simulink model "FighterAC"  (R2018a)
settings: Solver=ode2  StartTime=0.0  StopTime=T_final  FixedStep=dt_sim  RelTol=1e-3
undefined symbols (not defined in the file): b, Cl_da, Cl_dr, Cl_p, Cl_r, Cn_da, Cn_dr, Cn_p, Cn_r, Cy_da, Cy_dr, Cy_p, Cy_r, g, Ixx, Izz, mass, S_ref, V_ini
libraries: simulink_need_slupdate x4
settings Model: Creator=Can  LastModifiedBy=Can

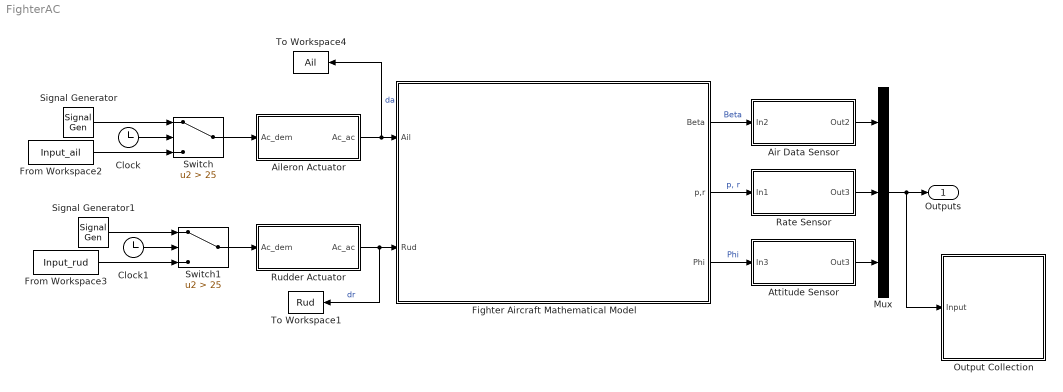
== system FighterAC ==
  Aileron Actuator : Subsystem
  Air Data Sensor : Subsystem
  Attitude Sensor : Subsystem
  Clock : Clock
  Clock1 : Clock
  Fighter Aircraft Mathematical Model : Subsystem
      mask Display: image('C:\Users\Can\Desktop\Thesis_v3\MMU.PNG')
  From Workspace2 : FromWorkspace  VariableName=Input_ail  SampleTime=0
  From Workspace3 : FromWorkspace  VariableName=Input_rud  SampleTime=0
  Mux : Mux  Inputs=3
  "Output Collection " : Subsystem
  Rate Sensor : Subsystem
  Rudder Actuator : Subsystem
  Signal Generator : SignalGenerator  WaveForm=square  Amplitude=0.05  Units=rad/sec
  Signal Generator1 : SignalGenerator  WaveForm=square  Amplitude=0.05  Units=rad/sec
  Switch : Switch  Criteria=u2 > Threshold  Threshold=25
  Switch1 : Switch  Criteria=u2 > Threshold  Threshold=25
  To Workspace1 : ToWorkspace  VariableName=Rud  SaveFormat=Structure With Time  SampleTime=-1
  To Workspace4 : ToWorkspace  VariableName=Ail  SaveFormat=Structure With Time  SampleTime=-1
  Outputs : Outport
  wires:
  From Workspace2/1 -> Switch/3
  Clock/1 -> Switch/2
  Signal Generator/1 -> Switch/1
  Signal Generator1/1 -> Switch1/1
  Clock1/1 -> Switch1/2
  From Workspace3/1 -> Switch1/3
  Attitude Sensor/1(Out3) -> Mux/3
  Air Data Sensor/1(Out2) -> Mux/1
  Fighter Aircraft Mathematical Model/3(Phi) -> Attitude Sensor/1(In3)  "Phi"
  Fighter Aircraft Mathematical Model/1(Beta) -> Air Data Sensor/1(In2)  "Beta"
  Rudder Actuator/1(Ac_ac) -> To Workspace1/1, Fighter Aircraft Mathematical Model/2(Rud)  "dr"
  Rate Sensor/1(Out3) -> Mux/2
  Mux/1 -> "Output Collection "/1(Input), Outputs/1
  Fighter Aircraft Mathematical Model/2(p,r) -> Rate Sensor/1(In1)  "p, r"
  Aileron Actuator/1(Ac_ac) -> To Workspace4/1, Fighter Aircraft Mathematical Model/1(Ail)  "da"
  Switch1/1 -> Rudder Actuator/1(Ac_dem)
  Switch/1 -> Aileron Actuator/1(Ac_dem)

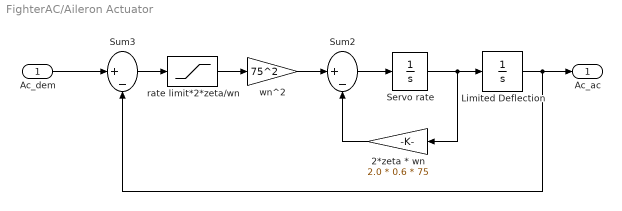
== system FighterAC/Aileron Actuator ==
  Ac_dem : Inport
  2*zeta * wn : Gain  Gain=2.0 * 0.6 * 75  SaturateOnIntegerOverflow=on  OutDataTypeStr=Inherit: Same as input  ParamDataTypeStr=Inherit: Same as input
  Limited Deflection : Integrator  LimitOutput=on  UpperSaturationLimit=25*pi/180  LowerSaturationLimit=-25*pi/180
  Servo rate : Integrator
  Sum2 : Sum  Inputs=|+-  SaturateOnIntegerOverflow=on  InputSameDT=on  OutDataTypeStr=Inherit: Same as first input
  Sum3 : Sum  Inputs=|+-  SaturateOnIntegerOverflow=on  InputSameDT=on  OutDataTypeStr=Inherit: Same as first input
  rate limit*2*zeta/wn : Saturate  UpperLimit=(80*pi/180)*2*0.6/75  LowerLimit=-(80*pi/180)*2*0.6/75
  wn^2 : Gain  Gain=75^2  SaturateOnIntegerOverflow=on  OutDataTypeStr=Inherit: Same as input  ParamDataTypeStr=Inherit: Same as input
  Ac_ac : Outport  InitialOutput=0
  wires:
  Limited Deflection/1 -> Ac_ac/1, Sum3/2
  2*zeta * wn/1 -> Sum2/2
  wn^2/1 -> Sum2/1
  Sum2/1 -> Servo rate/1
  Servo rate/1 -> 2*zeta * wn/1, Limited Deflection/1
  rate limit*2*zeta/wn/1 -> wn^2/1
  Ac_dem/1 -> Sum3/1
  Sum3/1 -> rate limit*2*zeta/wn/1

== system FighterAC/Air Data Sensor ==
  note: AIR DATA SENSOR
  In2 : Inport
  Air Data Sensor Dynamics : TransferFcn  Numerator=[0.116 -14.437 905.92]  Denominator=[1 29.573 908.77]
  Out2 : Outport
  wires:
  In2/1 -> Air Data Sensor Dynamics/1
  Air Data Sensor Dynamics/1 -> Out2/1

== system FighterAC/Attitude Sensor ==
  note: ATTITUDE SENSOR
  In3 : Inport
  Attitude Sensor Dynamics : TransferFcn  Numerator=[0.3417 -82.317 7161.8]  Denominator=[1 190.85 7162.3]
  Out3 : Outport
  wires:
  In3/1 -> Attitude Sensor Dynamics/1
  Attitude Sensor Dynamics/1 -> Out3/1

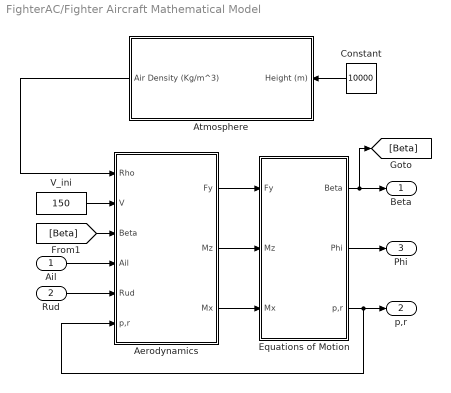
== system FighterAC/Fighter Aircraft Mathematical Model ==
  Ail : Inport
  Rud : Inport  Port=2
  Aerodynamics : Subsystem
  Atmosphere : Subsystem  AncestorBlock=aerospace/Atmosphere/Atmosphere model  mask(Atmosphere Model){}
      mask help: Compute International Standard Atmosphere (ISA) model for altitudes between 0 Km and 20 Km.
      mask init:
      | g=9.80665; % m/s
      | gamma = 1.4;
      | R = 287.0531; %J/Kg/K
      | L = 0.0065; % K/m
      | h_trop = 11000; % m
      | rho0 = 1.225; %Kg/m^3
      | P0 = 101325; % Pa
      | T0 = 288.15; % K
      mask Help:
      | <p>This block contains the International Standard Atmosphere (ISA) model for altitudes between 0 and 20 Km.  If the height input is greater than 20 Km, the height will be limited to 20 Km.</p>
      | 
      | <p><H4>Block Input</H4>
      | <ul>
      |     <li>Height - Altitude in meters</li>
      | </ul>
      | </p>
      | <p><H4>Block Outputs</H4>
      | <ul>
      |     <li>Temperature - in degree Kelvin</li>
      |     <li>Speed of Sound - in meters/second</li>
      |     <li>Air Pressure - in Pascals</li>
      |     <li>Air Density - in kilograms/meter</li>
      | </ul>
      | </p>
  Constant : Constant  Value=10000
  Equations of Motion : Subsystem
  V_ini : Constant  Value=150
  Beta : Outport  InitialOutput=0
  p,r : Outport  Port=2  InitialOutput=0
  Phi : Outport  Port=3  InitialOutput=0
  wires:
  Rud/1 -> Aerodynamics/5(Rud)
  [Beta] -> Aerodynamics/3(Beta)
  Aerodynamics/1(Fy) -> Equations of Motion/1(Fy)
  Aerodynamics/2(" Mz") -> Equations of Motion/2(Mz)
  Aerodynamics/3(" Mx") -> Equations of Motion/3(Mx)
  Equations of Motion/2(Phi) -> Phi/1
  Atmosphere/1(Air Density (Kg/m^3)) -> Aerodynamics/1(Rho)
  Ail/1 -> Aerodynamics/4(Ail)
  Constant/1 -> Atmosphere/1(Height (m))
  V_ini/1 -> Aerodynamics/2(V)
  Equations of Motion/3(p,r) -> p,r/1, Aerodynamics/6(p,r)
  Equations of Motion/1(Beta) -> [Beta], Beta/1

== system FighterAC/Output Collection  ==
  Input : Inport
  Demux : Demux
  To Workspace1 : ToWorkspace  VariableName=P  SaveFormat=Structure With Time  SampleTime=-1
  To Workspace2 : ToWorkspace  VariableName=Phi  SaveFormat=Structure With Time  SampleTime=-1
  To Workspace4 : ToWorkspace  VariableName=Beta  SaveFormat=Structure With Time  SampleTime=-1
  To Workspace6 : ToWorkspace  VariableName=R  SaveFormat=Structure With Time  SampleTime=-1
  wires:
  Input/1 -> Demux/1
  Demux/1 -> To Workspace4/1
  Demux/4 -> To Workspace2/1
  Demux/3 -> To Workspace6/1
  Demux/2 -> To Workspace1/1

== system FighterAC/Rate Sensor ==
  note: RATE SENSOR
  In1 : Inport
  Demux : Demux  Outputs=2
  Mux : Mux  Inputs=2
  Rate Sensor Dynamics : TransferFcn  Numerator=[0.00019 -0.0173 1]  Denominator=[0.000704 0.0401 1]
  Rate Sensor Dynamics2 : TransferFcn  Numerator=[0.00019 -0.0173 1]  Denominator=[0.000704 0.0401 1]
  Out3 : Outport
  wires:
  Demux/1 -> Rate Sensor Dynamics/1
  Demux/2 -> Rate Sensor Dynamics2/1
  In1/1 -> Demux/1
  Mux/1 -> Out3/1
  Rate Sensor Dynamics/1 -> Mux/1
  Rate Sensor Dynamics2/1 -> Mux/2

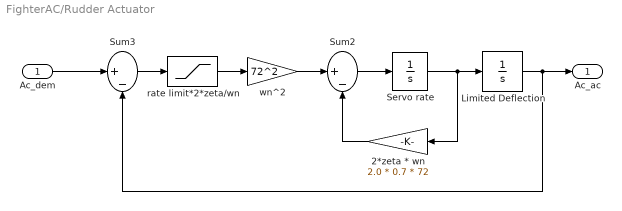
== system FighterAC/Rudder Actuator ==
  Ac_dem : Inport
  2*zeta * wn : Gain  Gain=2.0 * 0.7 * 72  SaturateOnIntegerOverflow=on  OutDataTypeStr=Inherit: Same as input  ParamDataTypeStr=Inherit: Same as input
  Limited Deflection : Integrator  LimitOutput=on  UpperSaturationLimit=30*pi/180  LowerSaturationLimit=-30*pi/180
  Servo rate : Integrator
  Sum2 : Sum  Inputs=|+-  SaturateOnIntegerOverflow=on  InputSameDT=on  OutDataTypeStr=Inherit: Same as first input
  Sum3 : Sum  Inputs=|+-  SaturateOnIntegerOverflow=on  InputSameDT=on  OutDataTypeStr=Inherit: Same as first input
  rate limit*2*zeta/wn : Saturate  UpperLimit=(120*pi/180)*2*0.7/72  LowerLimit=-(120*pi/180)*2*0.7/72
  wn^2 : Gain  Gain=72^2  SaturateOnIntegerOverflow=on  OutDataTypeStr=Inherit: Same as input  ParamDataTypeStr=Inherit: Same as input
  Ac_ac : Outport  InitialOutput=0
  wires:
  Ac_dem/1 -> Sum3/1
  rate limit*2*zeta/wn/1 -> wn^2/1
  Servo rate/1 -> 2*zeta * wn/1, Limited Deflection/1
  Sum2/1 -> Servo rate/1
  wn^2/1 -> Sum2/1
  Limited Deflection/1 -> Ac_ac/1, Sum3/2
  Sum3/1 -> rate limit*2*zeta/wn/1
  2*zeta * wn/1 -> Sum2/2

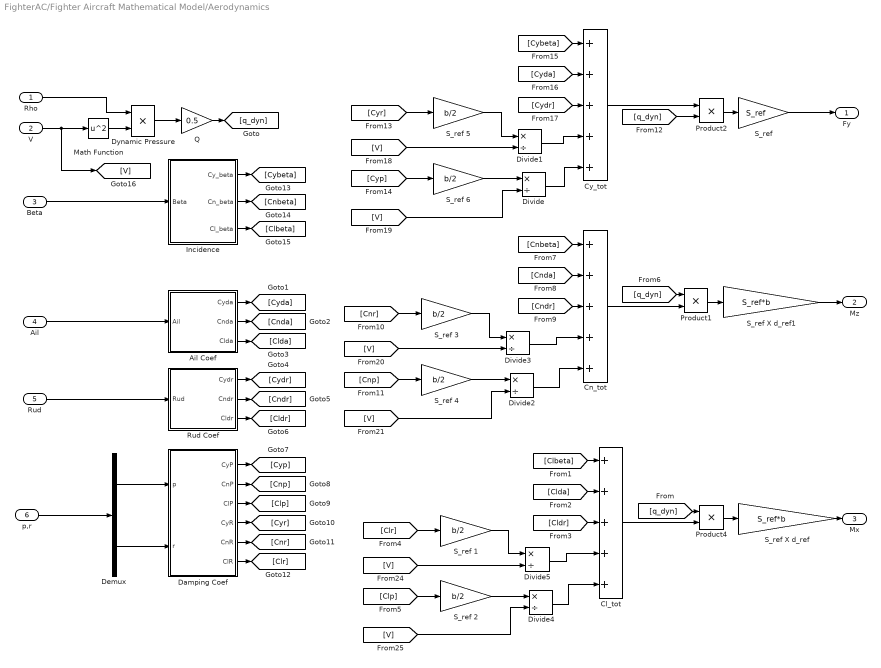
== system FighterAC/Fighter Aircraft Mathematical Model/Aerodynamics ==
  Rho : Inport
  V : Inport  Port=2
  Beta : Inport  Port=3
  Ail : Inport  Port=4
  Rud : Inport  Port=5
  p,r : Inport  Port=6
  Ail Coef : Subsystem
  Cl_tot : Sum  Inputs=+++++  SaturateOnIntegerOverflow=on  InputSameDT=on  OutDataTypeStr=Inherit: Same as first input
  Cn_tot : Sum  Inputs=+++++  SaturateOnIntegerOverflow=on  InputSameDT=on  OutDataTypeStr=Inherit: Same as first input
  Cy_tot : Sum  Inputs=+++++  SaturateOnIntegerOverflow=on  InputSameDT=on  OutDataTypeStr=Inherit: Same as first input
  Damping Coef : Subsystem
  Demux : Demux  Outputs=2
  Divide{,1..5} (6 alike) : Product  Inputs=*/
  Dynamic Pressure : Product  SaturateOnIntegerOverflow=on  InputSameDT=on  OutDataTypeStr=Inherit: Same as first input
  Incidence : Subsystem
  Math Function : Math  Operator=square  SaturateOnIntegerOverflow=on
  Product1 : Product  SaturateOnIntegerOverflow=on  InputSameDT=on  OutDataTypeStr=Inherit: Same as first input
  Product2 : Product  SaturateOnIntegerOverflow=on  InputSameDT=on  OutDataTypeStr=Inherit: Same as first input
  Product4 : Product  SaturateOnIntegerOverflow=on  InputSameDT=on  OutDataTypeStr=Inherit: Same as first input
  Q : Gain  Gain=0.5  SaturateOnIntegerOverflow=on  OutDataTypeStr=Inherit: Same as input  ParamDataTypeStr=Inherit: Same as input
  Rud Coef : Subsystem
  S_ref : Gain  Gain=S_ref  SaturateOnIntegerOverflow=on  OutDataTypeStr=Inherit: Same as input  ParamDataTypeStr=Inherit: Same as input
  S_ref {1..6} (6 alike) : Gain  Gain=b/2  SaturateOnIntegerOverflow=on  OutDataTypeStr=Inherit: Same as input  ParamDataTypeStr=Inherit: Same as input
  S_ref X d_ref : Gain  Gain=S_ref*b  SaturateOnIntegerOverflow=on  OutDataTypeStr=Inherit: Same as input  ParamDataTypeStr=Inherit: Same as input
  S_ref X d_ref1 : Gain  Gain=S_ref*b  SaturateOnIntegerOverflow=on  OutDataTypeStr=Inherit: Same as input  ParamDataTypeStr=Inherit: Same as input
  Fy : Outport  InitialOutput=[0]
  " Mz" : Outport  Port=2  InitialOutput=0
  " Mx" : Outport  Port=3  InitialOutput=0
  wires:
  Cl_tot/1 -> Product4/2
  Product4/1 -> S_ref X d_ref/1
  S_ref X d_ref/1 -> " Mx"/1
  Ail/1 -> Ail Coef/1(Ail)
  S_ref/1 -> Fy/1
  Product2/1 -> S_ref/1
  Cy_tot/1 -> Product2/1
  Beta/1 -> Incidence/1(Beta)
  V/1 -> [V], Math Function/1
  Dynamic Pressure/1 -> Q/1
  Rho/1 -> Dynamic Pressure/1
  Math Function/1 -> Dynamic Pressure/2
  Q/1 -> [q_dyn]
  [q_dyn] -> Product4/1
  [Clbeta] -> Cl_tot/1
  [Clda] -> Cl_tot/2
  [Cldr] -> Cl_tot/3
  Divide5/1 -> Cl_tot/4
  Divide4/1 -> Cl_tot/5
  Divide2/1 -> Cn_tot/5
  Divide3/1 -> Cn_tot/4
  [Cndr] -> Cn_tot/3
  [Cnda] -> Cn_tot/2
  [Cnbeta] -> Cn_tot/1
  [q_dyn] -> Product1/1
  S_ref X d_ref1/1 -> " Mz"/1
  Product1/1 -> S_ref X d_ref1/1
  Cn_tot/1 -> Product1/2
  [q_dyn] -> Product2/2
  [Cybeta] -> Cy_tot/1
  [Cyda] -> Cy_tot/2
  [Cyr] -> S_ref 5/1
  [Cyp] -> S_ref 6/1
  [Cydr] -> Cy_tot/3
  Rud/1 -> Rud Coef/1(Rud)
  Ail Coef/1(Cyda) -> [Cyda]
  Ail Coef/2(Cnda) -> [Cnda]
  Ail Coef/3(Clda) -> [Clda]
  Rud Coef/3(Cldr) -> [Cldr]
  Rud Coef/2(Cndr) -> [Cndr]
  Rud Coef/1(Cydr) -> [Cydr]
  Demux/1 -> Damping Coef/1(p)
  Demux/2 -> Damping Coef/2(r)
  Damping Coef/3(ClP) -> [Clp]
  Damping Coef/2(CnP) -> [Cnp]
  Damping Coef/1(CyP) -> [Cyp]
  Damping Coef/6(ClR) -> [Clr]
  Damping Coef/5(CnR) -> [Cnr]
  Damping Coef/4(CyR) -> [Cyr]
  Incidence/3(Cl_beta) -> [Clbeta]
  Incidence/2(Cn_beta) -> [Cnbeta]
  S_ref 6/1 -> Divide/1
  S_ref 5/1 -> Divide1/1
  Divide1/1 -> Cy_tot/4
  Divide/1 -> Cy_tot/5
  [V] -> Divide1/2
  [V] -> Divide/2
  [V] -> Divide2/2
  [V] -> Divide3/2
  S_ref 3/1 -> Divide3/1
  S_ref 4/1 -> Divide2/1
  [Cnp] -> S_ref 4/1
  [Cnr] -> S_ref 3/1
  [Clr] -> S_ref 1/1
  [Clp] -> S_ref 2/1
  S_ref 2/1 -> Divide4/1
  S_ref 1/1 -> Divide5/1
  [V] -> Divide5/2
  [V] -> Divide4/2
  p,r/1 -> Demux/1
  Incidence/1(Cy_beta) -> [Cybeta]

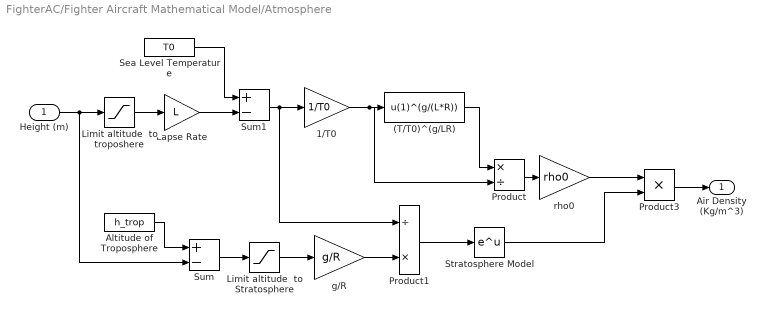
== system FighterAC/Fighter Aircraft Mathematical Model/Atmosphere ==
  Height (m) : Inport
  (T/T0)^(g/LR) : Fcn  Expr=u(1)^(g/(L*R))
  1/T0 : Gain  Gain=1/T0  SaturateOnIntegerOverflow=on  OutDataTypeStr=Inherit: Same as input  ParamDataTypeStr=Inherit: Same as input
  Altitude of Troposphere : Constant  Value=h_trop
  Lapse Rate : Gain  Gain=L  SaturateOnIntegerOverflow=on  OutDataTypeStr=Inherit: Same as input  ParamDataTypeStr=Inherit: Same as input
  Limit altitude  to Stratosphere : Saturate  UpperLimit=0  LowerLimit=h_trop-20000
  Limit altitude  to troposhere : Saturate  UpperLimit=h_trop  LowerLimit=0
  Product : Product  Inputs=*/  SaturateOnIntegerOverflow=on  RndMeth=Zero  InputSameDT=on  OutDataTypeStr=Inherit: Same as first input
  Product1 : Product  Inputs=/*  SaturateOnIntegerOverflow=on  RndMeth=Zero  InputSameDT=on  OutDataTypeStr=Inherit: Same as first input
  Product3 : Product  SaturateOnIntegerOverflow=on  RndMeth=Zero  InputSameDT=on  OutDataTypeStr=Inherit: Same as first input
  Sea Level Temperature : Constant  Value=T0
  Stratosphere Model : Math  SaturateOnIntegerOverflow=on
  Sum : Sum  Inputs=+-  SaturateOnIntegerOverflow=on  InputSameDT=on  OutDataTypeStr=Inherit: Same as first input
  Sum1 : Sum  Inputs=+-  SaturateOnIntegerOverflow=on  InputSameDT=on  OutDataTypeStr=Inherit: Same as first input
  g/R : Gain  Gain=g/R  SaturateOnIntegerOverflow=on  OutDataTypeStr=Inherit: Same as input  ParamDataTypeStr=Inherit: Same as input
  rho0 : Gain  Gain=rho0  SaturateOnIntegerOverflow=on  OutDataTypeStr=Inherit: Same as input  ParamDataTypeStr=Inherit: Same as input
  Air Density (Kg/m^3) : Outport  InitialOutput=0
  wires:
  Limit altitude  to Stratosphere/1 -> g/R/1
  Sum/1 -> Limit altitude  to Stratosphere/1
  Altitude of Troposphere/1 -> Sum/1
  Product1/1 -> Stratosphere Model/1
  g/R/1 -> Product1/2
  Stratosphere Model/1 -> Product3/2
  Product3/1 -> Air Density (Kg/m^3)/1
  rho0/1 -> Product3/1
  Sea Level Temperature/1 -> Sum1/1
  Lapse Rate/1 -> Sum1/2
  Sum1/1 -> Product1/1, 1/T0/1
  1/T0/1 -> Product/2, (T/T0)^(g/LR)/1
  (T/T0)^(g/LR)/1 -> Product/1
  Product/1 -> rho0/1
  Limit altitude  to troposhere/1 -> Lapse Rate/1
  Height (m)/1 -> Sum/2, Limit altitude  to troposhere/1

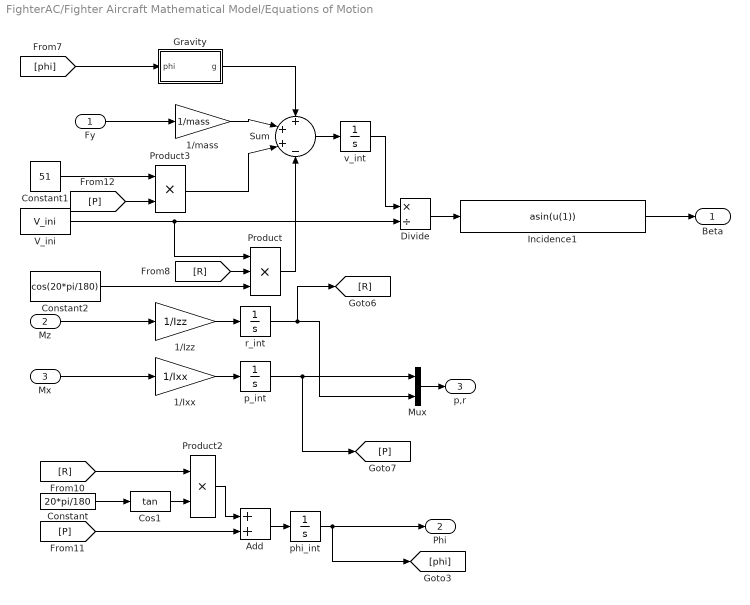
== system FighterAC/Fighter Aircraft Mathematical Model/Equations of Motion ==
  Fy : Inport
  Mz : Inport  Port=2
  Mx : Inport  Port=3
  1/Ixx : Gain  Gain=1/Ixx  SaturateOnIntegerOverflow=on  OutDataTypeStr=Inherit: Same as input  ParamDataTypeStr=Inherit: Same as input
  1/Izz : Gain  Gain=1/Izz  SaturateOnIntegerOverflow=on  OutDataTypeStr=Inherit: Same as input  ParamDataTypeStr=Inherit: Same as input
  1/mass : Gain  Gain=1/mass  SaturateOnIntegerOverflow=on  OutDataTypeStr=Inherit: Same as input  ParamDataTypeStr=Inherit: Same as input
  Add : Sum
  Constant : Constant  Value=20*pi/180
  Constant1 : Constant  Value=51
  Constant2 : Constant  Value=cos(20*pi/180)
  Cos1 : Trigonometry  Operator=tan
  Divide : Product  Inputs=*/
  Gravity : Subsystem
  Incidence1 : Fcn  Expr=asin(u(1))
  Mux : Mux  Inputs=2
  Product : Product  Inputs=3  SaturateOnIntegerOverflow=on  RndMeth=Zero  InputSameDT=on  OutDataTypeStr=Inherit: Same as first input
  Product2 : Product  SaturateOnIntegerOverflow=on  RndMeth=Zero  InputSameDT=on  OutDataTypeStr=Inherit: Same as first input
  Product3 : Product  SaturateOnIntegerOverflow=on  RndMeth=Zero  InputSameDT=on  OutDataTypeStr=Inherit: Same as first input
  Sum : Sum  Inputs=+++-  SaturateOnIntegerOverflow=on  InputSameDT=on  OutDataTypeStr=Inherit: Same as first input
  V_ini : Constant  Value=V_ini
  p_int : Integrator
  phi_int : Integrator  WrapState=on
  r_int : Integrator
  v_int : Integrator
  Beta : Outport  InitialOutput=0
  Phi : Outport  Port=2  InitialOutput=0
  p,r : Outport  Port=3  InitialOutput=0
  wires:
  [P] -> Add/2
  1/mass/1 -> Sum/2
  1/Ixx/1 -> p_int/1
  Gravity/1(g) -> Sum/1
  V_ini/1 -> Divide/2, Product/1
  Mx/1 -> 1/Ixx/1
  Product/1 -> Sum/4
  Sum/1 -> v_int/1
  Fy/1 -> 1/mass/1
  v_int/1 -> Divide/1
  Mz/1 -> 1/Izz/1
  1/Izz/1 -> r_int/1
  r_int/1 -> [R], Mux/2
  phi_int/1 -> [phi], Phi/1
  Add/1 -> phi_int/1
  Product2/1 -> Add/1
  Constant/1 -> Cos1/1
  Product3/1 -> Sum/3
  Constant1/1 -> Product3/1
  [P] -> Product3/2
  [phi] -> Gravity/1(phi)
  [R] -> Product/2
  [R] -> Product2/1
  p_int/1 -> Mux/1, [P]
  Cos1/1 -> Product2/2
  Divide/1 -> Incidence1/1
  Incidence1/1 -> Beta/1
  Constant2/1 -> Product/3
  Mux/1 -> p,r/1

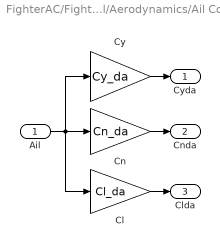
== system FighterAC/Fighter Aircraft Mathematical Model/Aerodynamics/Ail Coef ==
  Ail : Inport
  Cl : Gain  Gain=Cl_da  SaturateOnIntegerOverflow=on  OutDataTypeStr=Inherit: Same as input  ParamDataTypeStr=Inherit: Same as input
  Cn : Gain  Gain=Cn_da  SaturateOnIntegerOverflow=on  OutDataTypeStr=Inherit: Same as input  ParamDataTypeStr=Inherit: Same as input
  Cy : Gain  Gain=Cy_da  SaturateOnIntegerOverflow=on  OutDataTypeStr=Inherit: Same as input  ParamDataTypeStr=Inherit: Same as input
  Cyda : Outport  InitialOutput=0
  Cnda : Outport  Port=2  InitialOutput=0
  Clda : Outport  Port=3  InitialOutput=0
  wires:
  Cn/1 -> Cnda/1
  Cl/1 -> Clda/1
  Cy/1 -> Cyda/1
  Ail/1 -> Cy/1, Cn/1, Cl/1

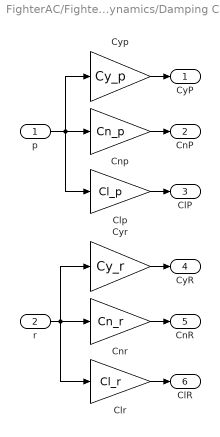
== system FighterAC/Fighter Aircraft Mathematical Model/Aerodynamics/Damping Coef ==
  p : Inport
  r : Inport  Port=2
  Clp : Gain  Gain=Cl_p  SaturateOnIntegerOverflow=on  OutDataTypeStr=Inherit: Same as input  ParamDataTypeStr=Inherit: Same as input
  Clr : Gain  Gain=Cl_r  SaturateOnIntegerOverflow=on  OutDataTypeStr=Inherit: Same as input  ParamDataTypeStr=Inherit: Same as input
  Cnp : Gain  Gain=Cn_p  SaturateOnIntegerOverflow=on  OutDataTypeStr=Inherit: Same as input  ParamDataTypeStr=Inherit: Same as input
  Cnr : Gain  Gain=Cn_r  SaturateOnIntegerOverflow=on  OutDataTypeStr=Inherit: Same as input  ParamDataTypeStr=Inherit: Same as input
  Cyp : Gain  Gain=Cy_p  SaturateOnIntegerOverflow=on  OutDataTypeStr=Inherit: Same as input  ParamDataTypeStr=Inherit: Same as input
  Cyr : Gain  Gain=Cy_r  SaturateOnIntegerOverflow=on  OutDataTypeStr=Inherit: Same as input  ParamDataTypeStr=Inherit: Same as input
  CyP : Outport  InitialOutput=0
  CnP : Outport  Port=2  InitialOutput=0
  ClP : Outport  Port=3  InitialOutput=0
  CyR : Outport  Port=4  InitialOutput=0
  CnR : Outport  Port=5  InitialOutput=0
  ClR : Outport  Port=6  InitialOutput=0
  wires:
  Cnp/1 -> CnP/1
  Clp/1 -> ClP/1
  Cyp/1 -> CyP/1
  p/1 -> Cyp/1, Cnp/1, Clp/1
  Cyr/1 -> CyR/1
  Clr/1 -> ClR/1
  Cnr/1 -> CnR/1
  r/1 -> Cyr/1, Clr/1, Cnr/1

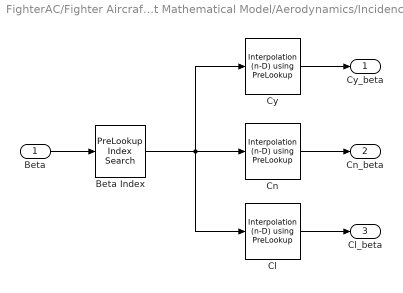
== system FighterAC/Fighter Aircraft Mathematical Model/Aerodynamics/Incidence ==
  Beta : Inport
  Beta Index : simulink_need_slupdate/PreLookup Index Search  bpData=beta  searchMode=Binary Search  cacheBpFlag=on  outputFlag=off  IndexDataType=uint32  extrapMode=Linear Extrapolation  rangeErrorMode=None
      settings: SourceProductName=Simulink  SourceProductBaseCode=SL
  Cl : simulink_need_slupdate/Interpolation (n-D) using PreLookup  numDimsPopupSelect=1  explicitNumDims=2  table=Cl_beta  interpMethod=Linear  extrapMethod=None - Clip  rangeErrorMode=None  NumSelectionDims=0
      settings: SourceProductName=Simulink  SourceProductBaseCode=SL
  Cn : simulink_need_slupdate/Interpolation (n-D) using PreLookup  numDimsPopupSelect=1  explicitNumDims=2  table=Cn_beta  interpMethod=Linear  extrapMethod=None - Clip  rangeErrorMode=None  NumSelectionDims=0
      settings: SourceProductName=Simulink  SourceProductBaseCode=SL
  Cy : simulink_need_slupdate/Interpolation (n-D) using PreLookup  numDimsPopupSelect=1  explicitNumDims=2  table=Cy_beta  interpMethod=Linear  extrapMethod=None - Clip  rangeErrorMode=None  NumSelectionDims=0
      settings: SourceProductName=Simulink  SourceProductBaseCode=SL
  Cy_beta : Outport  InitialOutput=0
  Cn_beta : Outport  Port=2  InitialOutput=0
  Cl_beta : Outport  Port=3  InitialOutput=0
  wires:
  Beta/1 -> Beta Index/1
  Cl/1 -> Cl_beta/1
  Cn/1 -> Cn_beta/1
  Cy/1 -> Cy_beta/1
  Beta Index/1 -> Cy/1, Cl/1, Cn/1

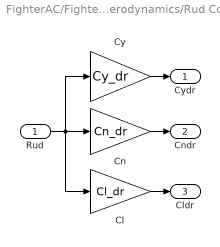
== system FighterAC/Fighter Aircraft Mathematical Model/Aerodynamics/Rud Coef ==
  Rud : Inport
  Cl : Gain  Gain=Cl_dr  SaturateOnIntegerOverflow=on  OutDataTypeStr=Inherit: Same as input  ParamDataTypeStr=Inherit: Same as input
  Cn : Gain  Gain=Cn_dr  SaturateOnIntegerOverflow=on  OutDataTypeStr=Inherit: Same as input  ParamDataTypeStr=Inherit: Same as input
  Cy : Gain  Gain=Cy_dr  SaturateOnIntegerOverflow=on  OutDataTypeStr=Inherit: Same as input  ParamDataTypeStr=Inherit: Same as input
  Cydr : Outport  InitialOutput=0
  Cndr : Outport  Port=2  InitialOutput=0
  Cldr : Outport  Port=3  InitialOutput=0
  wires:
  Rud/1 -> Cl/1, Cn/1, Cy/1
  Cy/1 -> Cydr/1
  Cl/1 -> Cldr/1
  Cn/1 -> Cndr/1

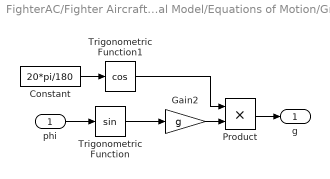
== system FighterAC/Fighter Aircraft Mathematical Model/Equations of Motion/Gravity ==
  phi : Inport
  Constant : Constant  Value=20*pi/180
  Gain2 : Gain  Gain=g  SaturateOnIntegerOverflow=on  OutDataTypeStr=Inherit: Same as input  ParamDataTypeStr=Inherit: Same as input
  Product : Product
  Trigonometric Function : Trigonometry
  Trigonometric Function1 : Trigonometry  Operator=cos
  g : Outport
  wires:
  phi/1 -> Trigonometric Function/1
  Trigonometric Function/1 -> Gain2/1
  Gain2/1 -> Product/2
  Product/1 -> g/1
  Trigonometric Function1/1 -> Product/1
  Constant/1 -> Trigonometric Function1/1
